simulink model "solar_photovoltaic_array"  (R2021a)
settings: Solver=FixedStepDiscrete  StartTime=1  StopTime=T.sim_tn  FixedStep=1  RelTol=1e-3
settings Model: Creator=user  LastModifiedBy=user
settings DataIOCC: SaveOutput=off  SignalLogging=off  DSMLogging=off  SaveTime=off  ReturnWorkspaceOutputs=off

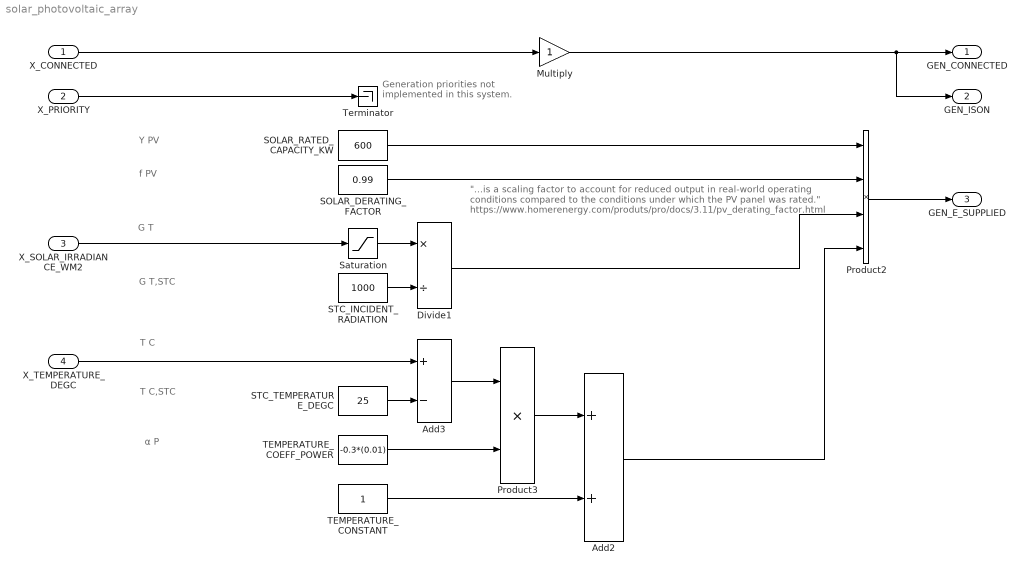
== system solar_photovoltaic_array ==
  note: Y PV
  note: Generation priorities
      | not implemented
      | in this system.
  note: "...is a scaling factor to account for reduced output in real-world operating
      | conditions compared to the conditions under which the PV panel was rated."
      | https://www.homerenergy.com/produts/pro/docs/3.11/pv_derating_factor.html
  note: f PV
  note: G T,STC
  note: T C,STC
  note: α P
  note: G T
  note: T C
  X_CONNECTED : Inport
  X_PRIORITY : Inport  Port=2
  X_SOLAR_IRRADIANCE_WM2 : Inport  Port=3
  X_TEMPERATURE_DEGC : Inport  Port=4
  Add2 : Sum
  Add3 : Sum  Inputs=+-
  Divide1 : Product  Inputs=*/
  Multiply : Gain
  Product2 : Product  Inputs=4
  Product3 : Product
  SOLAR_DERATING_FACTOR : Constant  Value=0.99
  SOLAR_RATED_CAPACITY_KW : Constant  Value=600
  STC_INCIDENT_RADIATION : Constant  Value=1000
  STC_TEMPERATURE_DEGC : Constant  Value=25
  Saturation : Saturate  UpperLimit=inf  LowerLimit=0
  TEMPERATURE_COEFF_POWER : Constant  Value=-0.3*(0.01)
  TEMPERATURE_CONSTANT : Constant
  Terminator : Terminator
  GEN_CONNECTED : Outport
  GEN_ISON : Outport  Port=2
  GEN_E_SUPPLIED : Outport  Port=3
  wires:
  Multiply/1 -> GEN_ISON/1, GEN_CONNECTED/1
  X_CONNECTED/1 -> Multiply/1
  X_PRIORITY/1 -> Terminator/1
  Product2/1 -> GEN_E_SUPPLIED/1
  SOLAR_RATED_CAPACITY_KW/1 -> Product2/1
  SOLAR_DERATING_FACTOR/1 -> Product2/2
  X_SOLAR_IRRADIANCE_WM2/1 -> Saturation/1
  STC_INCIDENT_RADIATION/1 -> Divide1/2
  Divide1/1 -> Product2/3
  X_TEMPERATURE_DEGC/1 -> Add3/1
  STC_TEMPERATURE_DEGC/1 -> Add3/2
  TEMPERATURE_COEFF_POWER/1 -> Product3/2
  Add3/1 -> Product3/1
  Product3/1 -> Add2/1
  TEMPERATURE_CONSTANT/1 -> Add2/2
  Add2/1 -> Product2/4
  Saturation/1 -> Divide1/1
